simulink model "assignment6"  (R2015a)
settings: Solver=ode45  StartTime=0.0  StopTime=3600  RelTol=1e-3
PreLoadFcn:
  | assignment5
values from neighbouring files (symbols this model uses):
  c = 1005.4    [assignment5(1).m]
  M = volumeHouse*airDensity    [assignment5(1).m]
  Mdot = flowrate*3600    (= 3600)    [assignment5(1).m]
  Rtot = 1/U_tot    [assignment5(1).m]
  TinIC = 20    [assignment5(1).m]
settings Model: Creator=kate  LastModifiedBy=kate

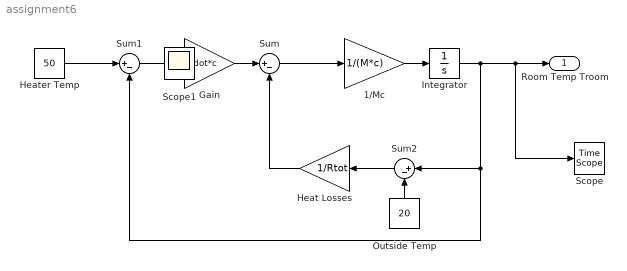
== system assignment6 ==
  "1/Mc " : Gain  Gain=1/(M*c)
  Gain : Gain  Gain=Mdot*c
  Heat Losses : Gain  Gain=1/Rtot
  "Heater Temp " : Constant  Value=50
  Integrator : Integrator  InitialCondition=TinIC
  "Outside Temp " : Constant  Value=20
  Scope : TimeScope
  Sum : Sum  Inputs=|+-
  Sum1 : Sum  Inputs=|+-
  Sum2 : Sum  Inputs=|+-
  "Room Temp Troom " : Outport
  Scope1 : Scope
  wires:
  Integrator/1 -> Sum2/1, Sum1/2, Scope/1, "Room Temp Troom "/1
  "1/Mc "/1 -> Integrator/1
  "Heater Temp "/1 -> Sum1/1
  Sum1/1 -> Gain/1
  Gain/1 -> Sum/1
  Sum/1 -> "1/Mc "/1
  "Outside Temp "/1 -> Sum2/2
  Sum2/1 -> Heat Losses/1
  Heat Losses/1 -> Sum/2
